simulink model "BLDC_Controller_2"  (R2024a)
settings: Solver=VariableStepAuto  StartTime=0.0  StopTime=1.5  RelTol=1e-3
libraries: spsThyristorLib x6, spsCurrentMeasurementLib x3, spsSeriesRLCBranchLib x2, eeBldcCurrentController x1, spsDCVoltageSourceLib x1, slpidlib x1, spsPermanentMagnetSynchronousMachineLib x1, sps_lib x1
settings Model: Creator=immor  LastModifiedBy=immor

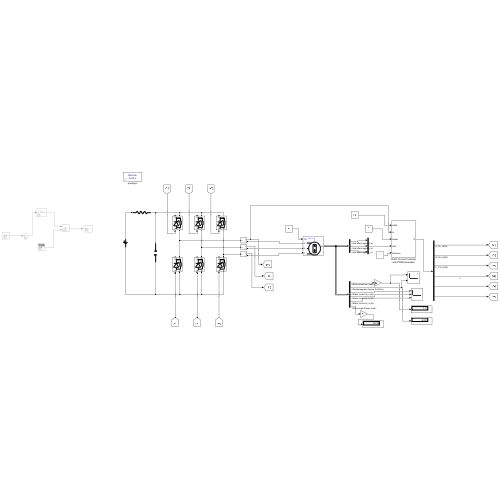
[thumbnail: Simulink's stored preview of the top-level diagram]
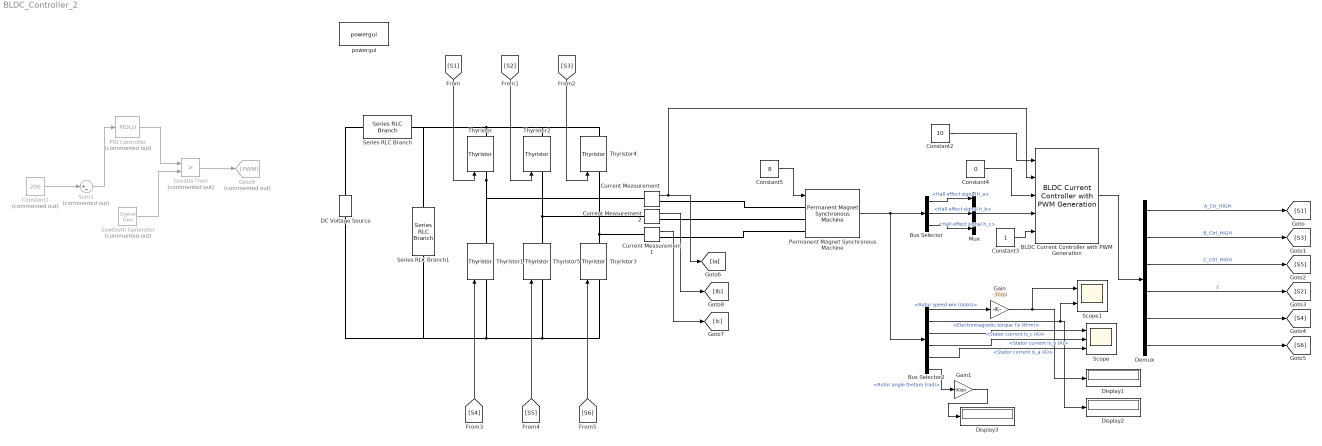
== system BLDC_Controller_2 ==
  BLDC Current Controller with PWM Generation : eeBldcCurrentController/BLDC Current Controller with PWM Generation  Kp=1  Ki=5  Kaw=1  Ts=-1  Tsd=0.001  ActZC=off  CarrCount=Up  Tper=0.001  Tfundamental=0.0001
      settings: LibrarySourceBlock=|
      | ee_sl_lib/BLDC Control/BLDC Current Controller
      | with PWM Generation
  Bus Selector : BusSelector  OutputSignals=Hall effect signal h_a,Hall effect signal h_b,Hall effect signal h_c
  Bus Selector2 : BusSelector  OutputSignals=Rotor speed wm (rad/s),Electromagnetic torque Te (N*m),Stator current is_c (A),Stator current is_b (A),Stator current is_a (A),Rotor angle thetam (rad)
  Constant1 : Constant  Commented=on  Value=200
  Constant2 : Constant  Value=10
  Constant3 : Constant
  Constant4 : Constant  Value=0
  Constant5 : Constant  Value=8
  Current Measurement : spsCurrentMeasurementLib/Current Measurement  PhasorSimulation=off  OutputType=Complex  PSBequivalent=0
  Current Measurement1 : spsCurrentMeasurementLib/Current Measurement  PhasorSimulation=off  OutputType=Complex  PSBequivalent=0
  Current Measurement2 : spsCurrentMeasurementLib/Current Measurement  PhasorSimulation=off  OutputType=Complex  PSBequivalent=0
  DC Voltage Source : spsDCVoltageSourceLib/DC Voltage Source  Amplitude=48  Measurements=None
  Demux : Demux  Outputs=6
  Display1 : Display
  Display2 : Display
  Display3 : Display
  Gain : Gain  Gain=-30/pi
  Gain1 : Gain  Gain=90/pi
  Goto9 : Goto  Commented=on  GotoTag=PWM
  GreaterThan : RelationalOperator  Commented=on  Operator=>  OutDataTypeStr=boolean  RndMeth=Simplest  InputSameDT=off
  Mux : Mux  Inputs=3
  PID Controller : slpidlib/PID Controller  Commented=on  Controller=PID  Form=Parallel  TimeDomain=Discrete-time  UseExternalTs=off  SampleTime=-1  IntegratorMethod=Forward Euler  FilterMethod=Forward Euler  ControllerParametersSource=internal  P=0.1  I=2  UseKiTs=off  D=0  UseExternalDerivativeSource=off  N=100  UseFilter=on  TunerSelectOption=Transfer Function Based (PID Tuner App)  InitialConditionSource=internal  InitialConditionForIntegrator=0  InitialConditionForFilter=0  DifferentiatorICPrevScaledInput=0  ExternalReset=none  TrackingMode=off  Kt=1  LimitOutput=off  SatLimitsSource=internal  UpperSaturationLimit=inf  LowerSaturationLimit=-inf  LinearizeAsGain=on  AntiWindupMode=none  Kb=1  LimitIntegrator=off  UpperIntegratorSaturationLimit=inf  LowerIntegratorSaturationLimit=-inf  POutMin=[]  POutMax=[]  IOutMin=[]  IOutMax=[]  DOutMin=[]  DOutMax=[]  NOutMin=[]  NOutMax=[]  SumOutMin=[]  SumOutMax=[]  SaturationOutMin=[]  SaturationOutMax=[]  PParamMin=[]  PParamMax=[]  IParamMin=[]  IParamMax=[]  DParamMin=[]  DParamMax=[]  NParamMin=[]  NParamMax=[]  KbParamMin=[]  KbParamMax=[]  KtParamMin=[]  KtParamMax=[]  KbOutMin=[]  KbOutMax=[]  KtOutMin=[]  KtOutMax=[]  IntegratorOutMin=[]  IntegratorOutMax=[]  FilterOutMin=[]  FilterOutMax=[]  SumI1OutMin=[]  SumI1OutMax=[]  SumI2OutMin=[]  SumI2OutMax=[]  SumI3OutMin=[]  SumI3OutMax=[]  SumI4OutMin=[]  SumI4OutMax=[]  SumDOutMin=[]  SumDOutMax=[]  DifferentiatorOutMin=[]  DifferentiatorOutMax=[]  FilterDiffOutCoefMin=[]  FilterDiffOutCoefMax=[]  ReciprocalOutMin=[]  ReciprocalOutMax=[]  SumDenOutMin=[]  SumDenOutMax=[]  SumNumOutMin=[]  SumNumOutMax=[]  DivideOutMin=[]  DivideOutMax=[]  UdiffTsProdOutMin=[]  UdiffTsProdOutMax=[]  NTsProdOutMin=[]  NTsProdOutMax=[]  UintegralTsProdOutMin=[]  UintegralTsProdOutMax=[]  UngainTsProdOutMin=[]  UngainTsProdOutMax=[]  ClampingZeroOutDataTypeStr=Inherit: Inherit via back propagation  ClampingZeroOutMin=[]  ClampingZeroOutMax=[]  FilterDenConstantOutDataTypeStr=Inherit: Inherit via back propagation  FilterDenConstantOutMin=[]  FilterDenConstantOutMax=[]  PCopyOutDataTypeStr=Inherit: Inherit via back propagation  PCopyOutMin=[]  PCopyOutMax=[]  NCopyOutDataTypeStr=Inherit: Inherit via back propagation  NCopyOutMin=[]  NCopyOutMax=[]  IntegratorContinuousStateAttributes=''  IntegratorStateMustResolveToSignalObject=off  IntegratorRTWStateStorageClass=Auto  FilterContinuousStateAttributes=''  FilterStateMustResolveToSignalObject=off  FilterRTWStateStorageClass=Auto  ParallelPVariant=InternalParameters  IdealPVariant=Disabled  IVariant=InternalParameters  DVariant=InternalParameters  IntegratorVariant=Discrete  SatVariant=Disabled  AWVariant=Passthrough  PCopyVariant=Disabled  TRVariant=Disabled  FdbkBlocksVariant=Forward  IdealPFdbkVariant=Disabled  SatFdbkVariant=Disabled  DerivativeFilterVariant=ForwardEulerFilter  NVariant=InternalParameters  NCopyVariant=Disabled  FilterICVariant=InternalICsFilter  IntegratorICVariant=InternalICs  ExternalResetVariant=Disabled  TRSumVariant=Passthrough  SumFdbkVariant=Disabled  SumVariant=Sum_PID  TsampFilterVariant=InternalTs  TsampNgainVariant=Passthrough  TsampIntegralVariant=Disabled_SignalSpec  ExternalSaturationOutDataTypeStr=Inherit: Same as second input  DerivativeSourceVariant=ErrorSignal
  Permanent Magnet Synchronous Machine : spsPermanentMagnetSynchronousMachineLib/Permanent Magnet Synchronous Machine  NbPhases=3  FluxDistribution=Sinusoidal  RotorType=Round  MechanicalLoad=Torque Tm  PresetModel=No  ShowDetailedParameters=on  MeasurementBus=off  Resistance=0.18  Inductance=8.5e-3  dqInductances=[8.5e-3,8.5e-3]  La=0.000835  MachineConstant=Flux linkage established by magnets (V.s)  Flux=10.1167  VoltageCst=7339.8656  TorqueCst=60.7002  Flat=120  Mechanical=[0.000621417 0.000303448 4]  PolePairs=4  InitialConditions=[0,0, 0,0]  InitialConditions5ph=[0 0 0 0 0 0]  RefAngle=90 degrees behind phase A axis (modified Park)  IterativeDiscreteModel=Trapezoidal non iterative  TsBlock=-1  TsPowergui=0
  Sawtooth Generator : SignalGenerator  Commented=on  WaveForm=sawtooth  Frequency=10000
  Scope : Scope  NumInputPorts=3
  Scope1 : Scope  NumInputPorts=2
  Series RLC Branch : spsSeriesRLCBranchLib/Series RLC Branch  LConnTagsString=__new0  RConnTagsString=__new0  BranchType=R  Resistance=3  Inductance=1e-3  SetiL0=off  InitialCurrent=0  Capacitance=1e-6  Setx0=off  InitialVoltage=0  Measurements=None
  Series RLC Branch1 : spsSeriesRLCBranchLib/Series RLC Branch  LConnTagsString=__new0  RConnTagsString=__new0  BranchType=C  Resistance=1  Inductance=1e-3  SetiL0=off  InitialCurrent=0  Capacitance=1e-3  Setx0=off  InitialVoltage=0  Measurements=None
  Sum1 : Sum  Commented=on  Inputs=|+-
  Thyristor{,1..5} (6 alike) : spsThyristorLib/Thyristor  Ron=0.001  Lon=0  Vf=0.8  IC=0  Rs=500  Cs=250e-9  Measurements=on
  powergui : sps_lib/powergui  Priority=1  SimulationMode=Discrete  SampleTime=1e-6  frequency=60  Iterations=50  frequencyindice=0  Pbase=100e6  ErrMax=1e-4  UnitsV=kV  UnitsW=MW  buscounter=0  FunctionMessages=off  echomessages=off  EnableUseOfTLC=off  CurrentSourceSwitches=off  DisableSnubberDevices=off  DisableRonSwitches=off  DisableVfSwitches=off  DisplayEquations=off  AutomaticDiscreteSolvers=off  SolverType=Tustin/Backward Euler (TBE)  Interpol=off  ExternalGateDelay=off  methode=off  Ts=100  x0status=blocks  SPID=on  SwTol=0  HookPort=off  NonlinearTolerance=1e-4  nMaxIteration=100  ContinueOnMaxIteration=off  RestoreLinks=warning  ResistiveCurrentMeasurement=off  Frange=[0:2:500]  Ylog=off  Xlog=on  ShowGrid=off  save=off  variable=ZData  structure=0  ZoomFFT=off  StartTime=0.0  cycles=1  DisplayStyle=1  fundamental=60  FreqAxis=off  MaxFrequency=1000  frequencyindicesteady=1  RmsSteady=1  display=off
  wires:
  Bus Selector/2 -> Mux/2  "<Hall effect signal h_b>"
  Bus Selector/3 -> Mux/3  "<Hall effect signal h_c>"
  Permanent Magnet Synchronous Machine/1 -> Bus Selector2/1, Bus Selector/1
  Current Measurement/1 -> BLDC Current Controller with PWM Generation/2, [Ia]
  Current Measurement1/1 -> [Ic]
  Current Measurement2/1 -> [Ib]
  Bus Selector2/1 -> Gain/1  "<Rotor speed wm (rad/s)>"
  Gain1/1 -> Display3/1
  Sawtooth Generator/1 -> GreaterThan/2
  Constant5/1 -> Permanent Magnet Synchronous Machine/1
  Constant1/1 -> Sum1/1
  Bus Selector/1 -> Mux/1  "<Hall effect signal h_a>"
  GreaterThan/1 -> Goto9/1
  Bus Selector2/2 -> Display2/1, Scope1/2  "<Electromagnetic torque Te (N*m)>"
  PID Controller/1 -> GreaterThan/1
  Gain/1 -> Scope1/1, Display1/1
  Bus Selector2/6 -> Gain1/1  "<Rotor angle thetam (rad)>"
  Sum1/1 -> PID Controller/1
  Mux/1 -> BLDC Current Controller with PWM Generation/4
  BLDC Current Controller with PWM Generation/1 -> Demux/1
  Constant2/1 -> BLDC Current Controller with PWM Generation/1
  Constant4/1 -> BLDC Current Controller with PWM Generation/3
  Constant3/1 -> BLDC Current Controller with PWM Generation/5
  Demux/1 -> [S1]  "A_Ctr_HIGH"
  Demux/2 -> [S3]  "B_Ctrl_HIGH"
  Demux/3 -> [S5]  "C_Ctrl_HIGH"
  Demux/4 -> [S2]  "z"
  Demux/5 -> [S4]
  Demux/6 -> [S6]
  [S1] -> Thyristor/1
  [S2] -> Thyristor2/1
  [S3] -> Thyristor4/1
  [S4] -> Thyristor1/1
  [S5] -> Thyristor5/1
  [S6] -> Thyristor3/1
  Bus Selector2/3 -> Scope/1  "<Stator current is_c (A)>"
  Bus Selector2/4 -> Scope/2  "<Stator current is_b (A)>"
  Bus Selector2/5 -> Scope/3  "<Stator current is_a (A)>"
  connections:
  Thyristor5/LConn1 -- DC Voltage Source/LConn1 -- Series RLC Branch1/RConn1 -- Thyristor1/LConn1 -- Thyristor3/LConn1
  Thyristor/RConn1 -- Thyristor2/RConn1 -- Thyristor4/RConn1 -- Series RLC Branch/RConn1 -- Series RLC Branch1/LConn1
  Current Measurement2/LConn1 -- Thyristor5/RConn1 -- Thyristor2/LConn1
  Thyristor/LConn1 -- Thyristor1/RConn1 -- Current Measurement/LConn1
  Current Measurement1/LConn1 -- Thyristor3/RConn1 -- Thyristor4/LConn1
  Current Measurement2/RConn1 -- Permanent Magnet Synchronous Machine/LConn2
  DC Voltage Source/RConn1 -- Series RLC Branch/LConn1
  Current Measurement1/RConn1 -- Permanent Magnet Synchronous Machine/LConn3
  Current Measurement/RConn1 -- Permanent Magnet Synchronous Machine/LConn1
